simulink library "sensor_gyroscope"  (R2025b)
settings: Solver=VariableStepAuto  StartTime=0.0  StopTime=10.0  RelTol=1e-3
values from neighbouring files (symbols this model uses):
  sens_gyro_D_bias_inst = 0.3 / 3600    (= 8.33333333333e-05)    [project_review.m]
  sens_gyro_D_RW = sens_gyro_RRW / sqrt(3600)    [project_review.m]
  sens_gyro_D_wn = sens_gyro_D_ARW / sqrt(3600)    [project_review.m]
  sens_gyro_O = [1,      sens_gyro_eps_xy, sens_gyro_eps_xz ... (first row only)    [project_review.m]
  sens_gyro_run_run_bias = 4 / 3600    (= 0.00111111111111)    [project_review.m]
  sens_gyro_SFE = 500 * 1e-6    (= 0.0005)    [project_review.m]
  sens_gyro_SFN = 15 * 1e-6    (= 1.5e-05)    [project_review.m]
  sens_gyro_static_temp_bias = 9 / 3600    (= 0.0025)    [project_review.m]
  sens_gyro_theta_eps = [0,            -sens_gyro_theta_eps_z,  sens_gyro_theta_eps_y ... (first row only)    [project_review.m]
  sens_gyro_Ts = 1 / sens_gyro_update_rate    (= 0.01)    [project_review.m]
undefined symbols (not defined in the file or in its folder): DiscIntNeverNeededParam
libraries: simulink_extras x1
settings Model: Creator=nicol  LastModifiedBy=User

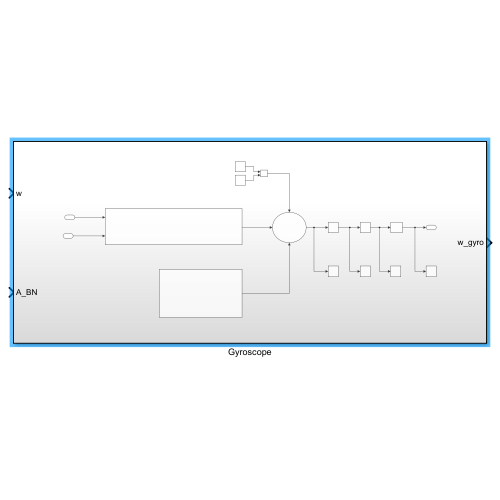
[thumbnail: Simulink's stored preview of the top-level diagram]
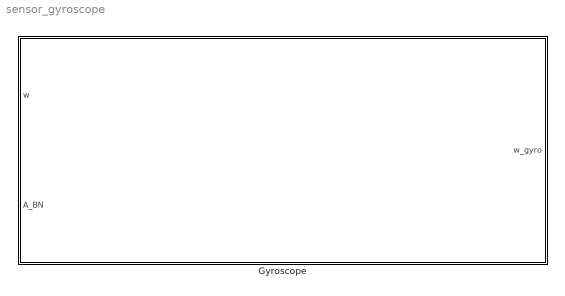
== system sensor_gyroscope ==
  Gyroscope : Subsystem

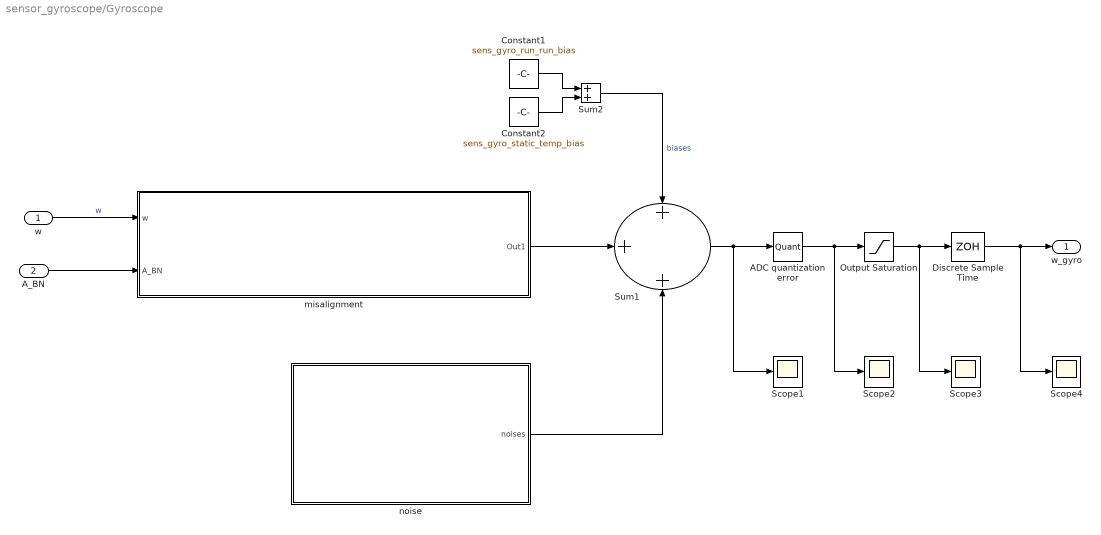
== system sensor_gyroscope/Gyroscope ==
  w : Inport
  A_BN : Inport  Port=2
  ADC quantization error : Quantizer  QuantizationInterval=sens_gyro_LSB
  Constant1 : Constant  Value=sens_gyro_run_run_bias
  Constant2 : Constant  Value=sens_gyro_static_temp_bias
  Discrete Sample Time : ZeroOrderHold  SampleTime=sens_gyro_Ts
  Output Saturation : Saturate  UpperLimit=20  LowerLimit=-20
  Scope{1..4} (4 alike) : Scope
      Scope1 settings: ActiveDisplayYMinimum=-0.032120647567430112  ActiveDisplayYMaximum=0.096644162809020939  DataLoggingVariableName=ScopeData2
      Scope2 settings: ActiveDisplayYMinimum=-1  ActiveDisplayYMaximum=1  DataLoggingVariableName=ScopeData3
      Scope3 settings: ActiveDisplayYMinimum=-1  ActiveDisplayYMaximum=1  DataLoggingVariableName=ScopeData4
      Scope4 settings: ActiveDisplayYMinimum=-0.032120647471039  ActiveDisplayYMaximum=0.096644162883216228  DataLoggingVariableName=ScopeData5
  Sum1 : Sum  Inputs=+++
  Sum2 : Sum
  misalignment : Subsystem
  noise : Subsystem
  w_gyro : Outport
  wires:
  Discrete Sample Time/1 -> w_gyro/1, Scope4/1
  Output Saturation/1 -> Discrete Sample Time/1, Scope3/1
  ADC quantization error/1 -> Output Saturation/1, Scope2/1
  Sum1/1 -> ADC quantization error/1, Scope1/1
  noise/1(noises) -> Sum1/3
  w/1 -> misalignment/1(w)  "w"
  A_BN/1 -> misalignment/2(A_BN)
  misalignment/1(Out1) -> Sum1/2
  Sum2/1 -> Sum1/1  "biases"
  Constant2/1 -> Sum2/2
  Constant1/1 -> Sum2/1

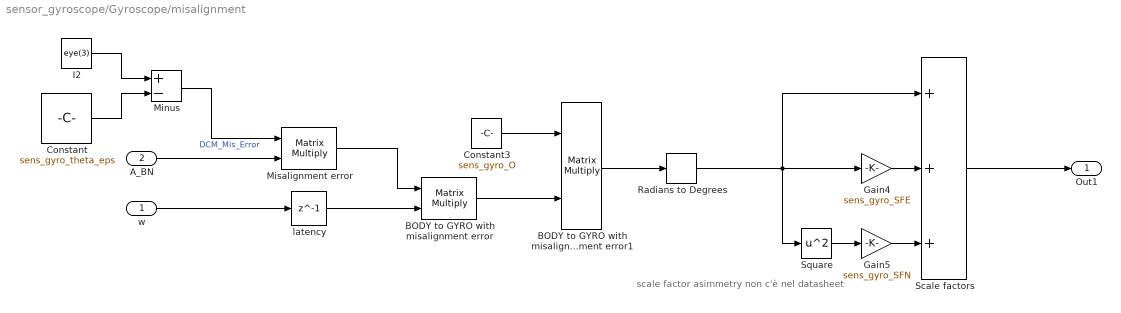
== system sensor_gyroscope/Gyroscope/misalignment ==
  note: scale factor asimmetry non c'è nel datasheet
  w : Inport
  A_BN : Inport  Port=2
  BODY to GYRO with misalignment error : Product  Multiplication=Matrix(*)
  BODY to GYRO with misalignment error1 : Product  Multiplication=Matrix(*)
  Constant : Constant  Value=sens_gyro_theta_eps
  Constant3 : Constant  Value=sens_gyro_O
  Gain4 : Gain  Gain=sens_gyro_SFE
  Gain5 : Gain  Gain=sens_gyro_SFN
  I2 : Constant  Value=eye(3)
  Minus : Sum  Inputs=+-
  Misalignment error : Product  Multiplication=Matrix(*)
  Radians to Degrees : simulink_extras/Transformations/Radians to Degrees
  Scale factors : Sum  Inputs=+++
  Square : Math  Operator=square
  latency : Delay  DelayLength=1
  Out1 : Outport
  wires:
  latency/1 -> BODY to GYRO with misalignment error/2
  BODY to GYRO with misalignment error/1 -> BODY to GYRO with misalignment error1/2
  Minus/1 -> Misalignment error/1  "DCM_Mis_Error"
  I2/1 -> Minus/1
  Radians to Degrees/1 -> Square/1, Gain4/1, Scale factors/1
  BODY to GYRO with misalignment error1/1 -> Radians to Degrees/1
  Misalignment error/1 -> BODY to GYRO with misalignment error/1
  A_BN/1 -> Misalignment error/2
  Gain5/1 -> Scale factors/3
  Constant/1 -> Minus/2
  w/1 -> latency/1
  Square/1 -> Gain5/1
  Constant3/1 -> BODY to GYRO with misalignment error1/1
  Gain4/1 -> Scale factors/2
  Scale factors/1 -> Out1/1

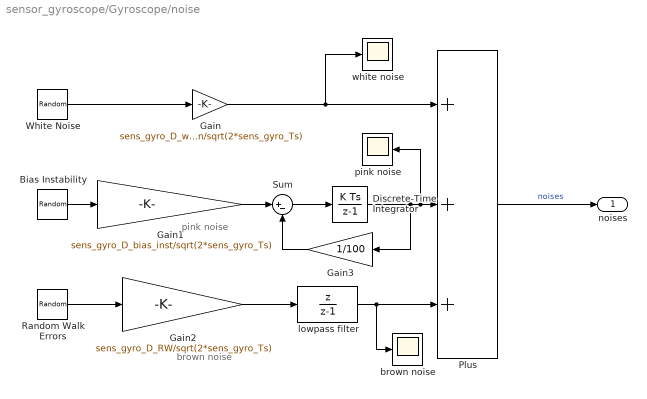
== system sensor_gyroscope/Gyroscope/noise ==
  note: brown noise
  note: pink noise
  " White Noise" : RandomNumber  SampleTime=0.1
  Bias Instability : RandomNumber  SampleTime=0.1
  Discrete-Time Integrator : DiscreteIntegrator  ICPrevOutput=DiscIntNeverNeededParam  ICPrevScaledInput=DiscIntNeverNeededParam
  Gain : Gain  Gain=sens_gyro_D_wn/sqrt(2*sens_gyro_Ts)
  Gain1 : Gain  Gain=sens_gyro_D_bias_inst/sqrt(2*sens_gyro_Ts)
  Gain2 : Gain  Gain=sens_gyro_D_RW/sqrt(2*sens_gyro_Ts)
  Gain3 : Gain  Gain=1/100
  Plus : Sum  Inputs=+++
  Random Walk Errors : RandomNumber  SampleTime=0.1
  Sum : Sum  Inputs=|+-
  brown noise : Scope
      settings: ActiveDisplayYMinimum=-0.025691906984189852  ActiveDisplayYMaximum=0.0025755592198982418  DataLoggingVariableName=ScopeData10
  lowpass filter : DiscreteTransferFcn  Numerator=[1 0]  Denominator=[1 -1]
  pink noise : Scope
      settings: ActiveDisplayYMinimum=-0.013777619312277414  ActiveDisplayYMaximum=0.014220901201123974  DataLoggingVariableName=ScopeData9
  white noise : Scope
      settings: ActiveDisplayYMinimum=-0.0017013348354620785  ActiveDisplayYMaximum=0.001720930099973718  DataLoggingVariableName=ScopeData8
  noises : Outport
  wires:
  " White Noise"/1 -> Gain/1
  Sum/1 -> Discrete-Time Integrator/1
  Gain3/1 -> Sum/2
  Gain2/1 -> lowpass filter/1
  Gain/1 -> Plus/1, white noise/1
  Discrete-Time Integrator/1 -> Gain3/1, Plus/2, pink noise/1
  Random Walk Errors/1 -> Gain2/1
  lowpass filter/1 -> brown noise/1, Plus/3
  Gain1/1 -> Sum/1
  Bias Instability/1 -> Gain1/1
  Plus/1 -> noises/1  "noises"
